simulink model "APPL_DriverFaultDetection"  (R2018b)
settings: configuration reference "CodeConfig_10_ms" (kept outside this file)
undefined symbols (not defined in the file): CAL_LockErrNoTime_30ms, CAL_ManualSwValid_90s, CAL_MotorHallInvalid_2s, CAL_MotorMaxRunTime_60s, CAL_MotorRelayErr_2s, CAL_MotorStall_750ms, D_DrSoftStopDef_B, D_DrSoftStopDef_F, D_DrSoftStopDef_H, D_DrSoftStopDef_L, D_Relay_DownBackFault, D_Relay_UpFrontFault, enSeatMoveCmd, FALSE, TRUE
libraries: DareLib x95, simulink x2
(part 1 of 3)
settings Model: Creator=Administrator  LastModifiedBy=Administrator
settings ConfigSetRef: SourceLocation=Base Workspace

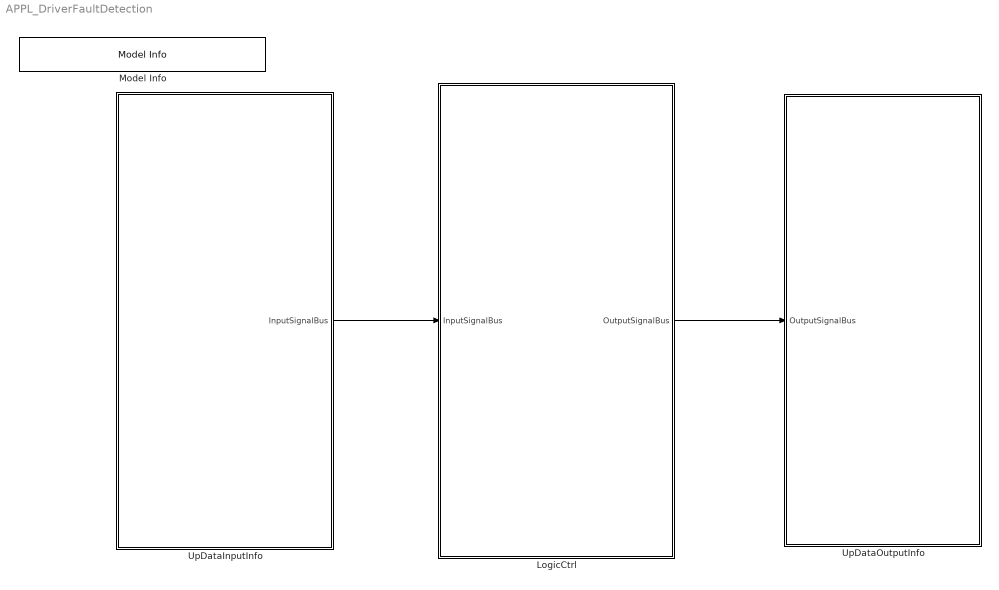
== system APPL_DriverFaultDetection ==
  LogicCtrl : Subsystem
  Model Info : simulink/Model-Wide Utilities/Model Info  Frame=on  DisplayStringWithTags=Version：%<ModelVersion>  HorizontalTextAlignment=Center  LeftAlignmentValue=0.5
  UpDataInputInfo : Subsystem  Priority=0  TreatAsAtomicUnit=on  RTWFileName=WiperCtrl
      settings: RTWSystemCode=Nonreusable function  RTWFcnNameOpts=Use subsystem name
  UpDataOutputInfo : Subsystem  Priority=2  TreatAsAtomicUnit=on  RTWFileName=WiperCtrl
      settings: RTWSystemCode=Nonreusable function  RTWFcnNameOpts=Use subsystem name
  wires:
  UpDataInputInfo/1(InputSignalBus) -> LogicCtrl/1(InputSignalBus)
  LogicCtrl/1(OutputSignalBus) -> UpDataOutputInfo/1(OutputSignalBus)

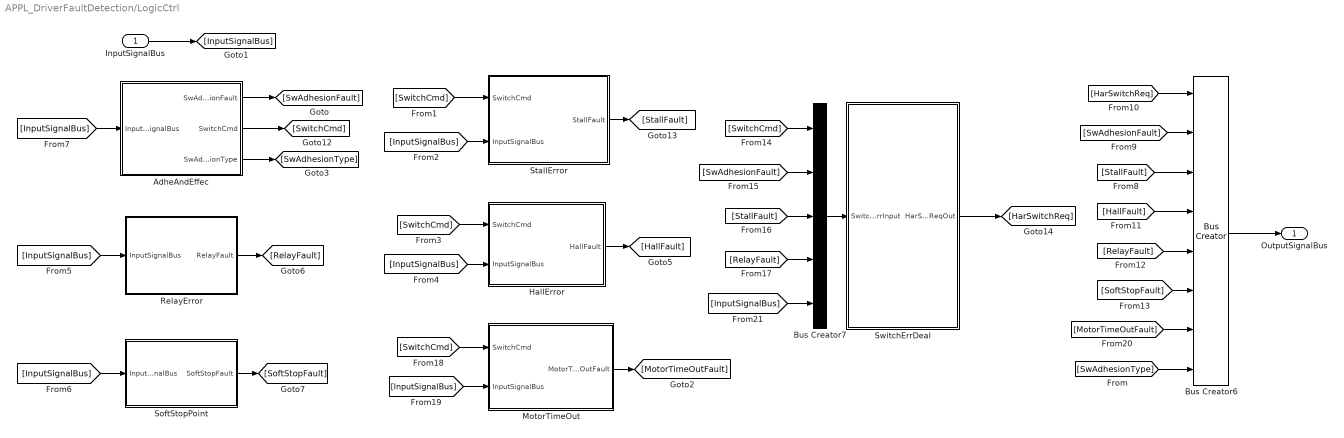
== system APPL_DriverFaultDetection/LogicCtrl ==
  InputSignalBus : Inport
  AdheAndEffec : Subsystem  Description=硬线开关粘连与有效检测
      settings: AttributesFormatString=%<Description>
  Bus Creator6 : BusCreator  Inputs=8
  Bus Creator7 : BusCreator  Inputs=5
  HallError : Subsystem  Description=电机霍尔故障检测
      settings: AttributesFormatString=%<Description>
  MotorTimeOut : Subsystem  Description=电机运行超时检测
      settings: AttributesFormatString=%<Description>
  RelayError : Subsystem  Description=继电器粘连故障检测
      settings: AttributesFormatString=%<Description>
  SoftStopPoint : Subsystem  Description=软止点检测
      settings: AttributesFormatString=%<Description>
  StallError : Subsystem  Description=电机堵转故障检测
      settings: AttributesFormatString=%<Description>
  SwitchErrDeal : Subsystem  Description=硬线开关故障处理
      settings: AttributesFormatString=%<Description>
  OutputSignalBus : Outport
  wires:
  InputSignalBus/1 -> [InputSignalBus]
  [StallFault] -> Bus Creator6/3
  [HallFault] -> Bus Creator6/4
  [SwAdhesionFault] -> Bus Creator6/2
  [RelayFault] -> Bus Creator6/5
  [HarSwitchReq] -> Bus Creator6/1
  [SoftStopFault] -> Bus Creator6/6
  Bus Creator6/1 -> OutputSignalBus/1
  [InputSignalBus] -> AdheAndEffec/1(InputSignalBus)
  AdheAndEffec/1(SwAdhesionFault) -> [SwAdhesionFault]
  AdheAndEffec/2(SwitchCmd) -> [SwitchCmd]
  [SwitchCmd] -> StallError/1(SwitchCmd)
  [InputSignalBus] -> StallError/2(InputSignalBus)
  StallError/1(StallFault) -> [StallFault]
  [SwitchCmd] -> HallError/1(SwitchCmd)
  [InputSignalBus] -> HallError/2(InputSignalBus)
  HallError/1(HallFault) -> [HallFault]
  [InputSignalBus] -> RelayError/1(InputSignalBus)
  RelayError/1(RelayFault) -> [RelayFault]
  SoftStopPoint/1(SoftStopFault) -> [SoftStopFault]
  [InputSignalBus] -> SoftStopPoint/1(InputSignalBus)
  SwitchErrDeal/1(HarSwitchReqOut) -> [HarSwitchReq]
  [SwitchCmd] -> Bus Creator7/1
  [StallFault] -> Bus Creator7/3
  [RelayFault] -> Bus Creator7/4
  [SwAdhesionFault] -> Bus Creator7/2
  Bus Creator7/1 -> SwitchErrDeal/1(SwitchErrInput)
  [SwitchCmd] -> MotorTimeOut/1(SwitchCmd)
  [InputSignalBus] -> MotorTimeOut/2(InputSignalBus)
  MotorTimeOut/1(MotorTimeOutFault) -> [MotorTimeOutFault]
  [MotorTimeOutFault] -> Bus Creator6/7
  [InputSignalBus] -> Bus Creator7/5
  AdheAndEffec/3(SwAdhesionType) -> [SwAdhesionType]
  [SwAdhesionType] -> Bus Creator6/8

== system APPL_DriverFaultDetection/UpDataInputInfo ==
  InputSignalProcess : Subsystem  Description=数据处理
      settings: AttributesFormatString=%<Description>  RTWSystemCode=Nonreusable function  RTWFcnNameOpts=Use subsystem name
  RTE_InputSignal : Subsystem  Description=接口自动生成  TreatAsAtomicUnit=on
      settings: AttributesFormatString=%<Description>  RTWSystemCode=Nonreusable function  RTWFcnNameOpts=Use subsystem name
  InputSignalBus : Outport
  wires:
  RTE_InputSignal/1(RTE_SignalBus) -> InputSignalProcess/1(RTE_SignalBus)
  InputSignalProcess/1(InputSignalBus) -> InputSignalBus/1  "InputSignalBus"

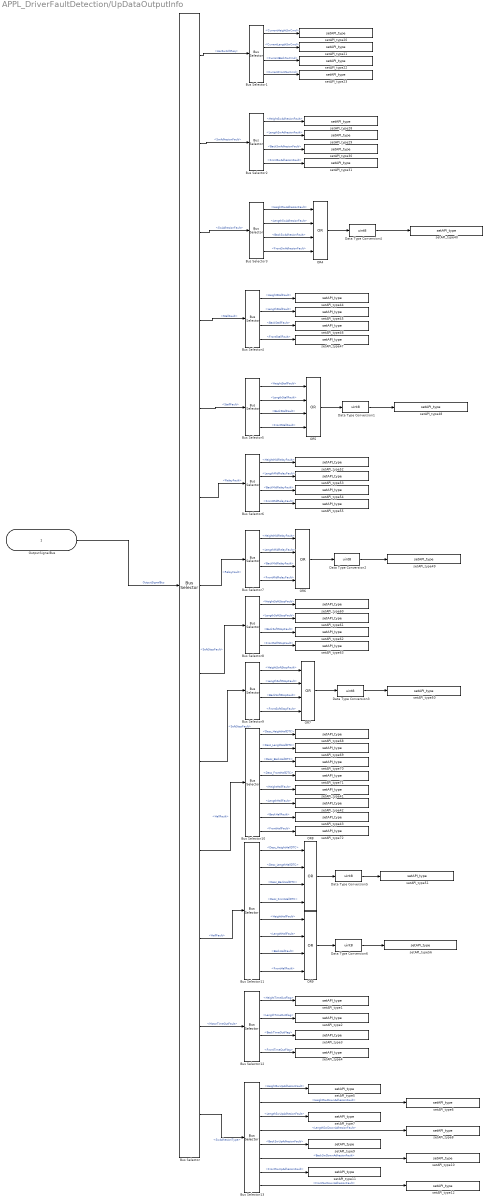
== system APPL_DriverFaultDetection/UpDataOutputInfo ==
  OutputSignalBus : Inport
  Bus Selector : BusSelector  OutputSignals=HarSwitchReq,SwAdhesionFault,SwAdhesionFault,StallFault,StallFault,RelayFault,RelayFault,SoftStopFault,SoftStopFault,HallFault,HallFault,MotorTimeOutFault,SwAdhesionType
  Bus Selector1 : BusSelector  OutputSignals=CurrentHeightSwCmd,CurrentLengthSwCmd,CurrentBackSwCmd,CurrentFrontSwCmd
  Bus Selector10 : BusSelector  OutputSignals=Desc_HeightHallDTC,Desc_LengthHallDTC,Desc_BackHallDTC,Desc_FrontHallDTC,HeightHallFault,LengthHallFault,BackHallFault,FrontHallFault
  Bus Selector11 : BusSelector  OutputSignals=Desc_HeightHallDTC,Desc_LengthHallDTC,Desc_BackHallDTC,Desc_FrontHallDTC,HeightHallFault,LengthHallFault,BackHallFault,FrontHallFault
  Bus Selector12 : BusSelector  OutputSignals=HeightTimeOutFlag,LengthTimeOutFlag,BackTimeOutFlag,FrontTimeOutFlag
  Bus Selector13 : BusSelector  OutputSignals=HeightSwUpAdhesionFault,HeightSwDownAdhesionFault,LengthSwUpAdhesionFault,LengthSwDownAdhesionFault,BackSwUpAdhesionFault,BackSwDownAdhesionFault,FrontSwUpAdhesionFault,FrontSwDownAdhesionFault
  Bus Selector2 : BusSelector  OutputSignals=HeightSwAdhesionFault,LengthSwAdhesionFault,BackSwAdhesionFault,FrontSwAdhesionFault
  Bus Selector3 : BusSelector  OutputSignals=HeightSwAdhesionFault,LengthSwAdhesionFault,BackSwAdhesionFault,FrontSwAdhesionFault
  Bus Selector4 : BusSelector  OutputSignals=HeightStallFault,LengthStallFault,BackStallFault,FrontStallFault
  Bus Selector5 : BusSelector  OutputSignals=HeightStallFault,LengthStallFault,BackStallFault,FrontStallFault
  Bus Selector6 : BusSelector  OutputSignals=HeightMidRelayFault,LengthMidRelayFault,BackMidRelayFault,FrontMidRelayFault
  Bus Selector7 : BusSelector  OutputSignals=HeightMidRelayFault,LengthMidRelayFault,BackMidRelayFault,FrontMidRelayFault
  Bus Selector8 : BusSelector  OutputSignals=HeightSoftStopFault,LengthSoftStopFault,BackSoftStopFault,FrontSoftStopFault
  Bus Selector9 : BusSelector  OutputSignals=HeightSoftStopFault,LengthSoftStopFault,BackSoftStopFault,FrontSoftStopFault
  Data Type Conversion{1..6} (6 alike) : DataTypeConversion  OutDataTypeStr=uint8
  OR{4..9} (6 alike) : Logic  Operator=OR  Inputs=4  AllPortsSameDT=off  OutDataTypeStr=boolean
  setAPI_type1 : DareLib/Dare/setAPI_type  g_funcname=Rte_SetVfb_DrHeightMotorTimeOutErr  g_param=""  g_type=uint8  g_size=-1
      settings: AttributesFormatString=%<g_funcname>  SourceProductName=Dare Library
  setAPI_type10 : DareLib/Dare/setAPI_type  g_funcname=Rte_SetVfb_DrBackSwitchAdheErr_Back  g_param=""  g_type=uint8  g_size=-1
      settings: AttributesFormatString=%<g_funcname>  SourceProductName=Dare Library
  setAPI_type11 : DareLib/Dare/setAPI_type  g_funcname=Rte_SetVfb_DrFrontSwitchAdheErr_ForWard  g_param=""  g_type=uint8  g_size=-1
      settings: AttributesFormatString=%<g_funcname>  SourceProductName=Dare Library
  setAPI_type12 : DareLib/Dare/setAPI_type  g_funcname=Rte_SetVfb_DrFrontSwitchAdheErr_Back  g_param=""  g_type=uint8  g_size=-1
      settings: AttributesFormatString=%<g_funcname>  SourceProductName=Dare Library
  setAPI_type2 : DareLib/Dare/setAPI_type  g_funcname=Rte_SetVfb_DrLengthMotorTimeOutErr  g_param=""  g_type=uint8  g_size=-1
      settings: AttributesFormatString=%<g_funcname>  SourceProductName=Dare Library
  setAPI_type20 : DareLib/Dare/setAPI_type  g_funcname=Rte_SetVfb_DrHeightSwitchCmd  g_param=""  g_type=uint8  g_enum=enSeatMoveCmd  g_size=-1
      settings: AttributesFormatString=%<g_funcname>  SourceProductName=Dare Library
  setAPI_type21 : DareLib/Dare/setAPI_type  g_funcname=Rte_SetVfb_DrLengthSwitchCmd  g_param=""  g_type=uint8  g_enum=enSeatMoveCmd  g_size=-1
      settings: AttributesFormatString=%<g_funcname>  SourceProductName=Dare Library
  setAPI_type22 : DareLib/Dare/setAPI_type  g_funcname=Rte_SetVfb_DrBackSwitchCmd  g_param=""  g_type=uint8  g_enum=enSeatMoveCmd  g_size=-1
      settings: AttributesFormatString=%<g_funcname>  SourceProductName=Dare Library
  setAPI_type23 : DareLib/Dare/setAPI_type  g_funcname=Rte_SetVfb_DrFrontSwitchCmd  g_param=""  g_type=uint8  g_enum=enSeatMoveCmd  g_size=-1
      settings: AttributesFormatString=%<g_funcname>  SourceProductName=Dare Library
  setAPI_type28 : DareLib/Dare/setAPI_type  g_funcname=Rte_SetVfb_DrHeightSwitchAdheErr  g_param=""  g_type=uint8  g_size=-1
      settings: AttributesFormatString=%<g_funcname>  SourceProductName=Dare Library
  setAPI_type29 : DareLib/Dare/setAPI_type  g_funcname=Rte_SetVfb_DrLengthSwitchAdheErr  g_param=""  g_type=uint8  g_size=-1
      settings: AttributesFormatString=%<g_funcname>  SourceProductName=Dare Library
  setAPI_type3 : DareLib/Dare/setAPI_type  g_funcname=Rte_SetVfb_DrBackMotorTimeOutErr  g_param=""  g_type=uint8  g_size=-1
      settings: AttributesFormatString=%<g_funcname>  SourceProductName=Dare Library
  setAPI_type30 : DareLib/Dare/setAPI_type  g_funcname=Rte_SetVfb_DrBackSwitchAdheErr  g_param=""  g_type=uint8  g_size=-1
      settings: AttributesFormatString=%<g_funcname>  SourceProductName=Dare Library
  setAPI_type31 : DareLib/Dare/setAPI_type  g_funcname=Rte_SetVfb_DrFrontSwitchAdheErr  g_param=""  g_type=uint8  g_size=-1
      settings: AttributesFormatString=%<g_funcname>  SourceProductName=Dare Library
  setAPI_type4 : DareLib/Dare/setAPI_type  g_funcname=Rte_SetVfb_DrFrontMotorTimeOutErr  g_param=""  g_type=uint8  g_size=-1
      settings: AttributesFormatString=%<g_funcname>  SourceProductName=Dare Library
  setAPI_type40 : DareLib/Dare/setAPI_type  g_funcname=Rte_SetVfb_DrAnyoneSwitchAdheErr  g_param=""  g_type=uint8  g_size=-1
      settings: AttributesFormatString=%<g_funcname>  SourceProductName=Dare Library
  setAPI_type41 : DareLib/Dare/setAPI_type  g_funcname=Rte_SetVfb_DrHeightHallErr  g_param=""  g_type=uint8  g_size=-1
      settings: AttributesFormatString=%<g_funcname>  SourceProductName=Dare Library
  setAPI_type42 : DareLib/Dare/setAPI_type  g_funcname=Rte_SetVfb_DrLengthHallErr  g_param=""  g_type=uint8  g_size=-1
      settings: AttributesFormatString=%<g_funcname>  SourceProductName=Dare Library
  setAPI_type43 : DareLib/Dare/setAPI_type  g_funcname=Rte_SetVfb_DrBackHallErr  g_param=""  g_type=uint8  g_size=-1
      settings: AttributesFormatString=%<g_funcname>  SourceProductName=Dare Library
  setAPI_type44 : DareLib/Dare/setAPI_type  g_funcname=Rte_SetVfb_DrHeightStallErr  g_param=""  g_type=uint8  g_size=-1
      settings: AttributesFormatString=%<g_funcname>  SourceProductName=Dare Library
  setAPI_type45 : DareLib/Dare/setAPI_type  g_funcname=Rte_SetVfb_DrLengthStallErr  g_param=""  g_type=uint8  g_size=-1
      settings: AttributesFormatString=%<g_funcname>  SourceProductName=Dare Library
  setAPI_type46 : DareLib/Dare/setAPI_type  g_funcname=Rte_SetVfb_DrBackStallErr  g_param=""  g_type=uint8  g_size=-1
      settings: AttributesFormatString=%<g_funcname>  SourceProductName=Dare Library
  setAPI_type47 : DareLib/Dare/setAPI_type  g_funcname=Rte_SetVfb_DrFrontStallErr  g_param=""  g_type=uint8  g_size=-1
      settings: AttributesFormatString=%<g_funcname>  SourceProductName=Dare Library
  setAPI_type48 : DareLib/Dare/setAPI_type  g_funcname=Rte_SetVfb_DrAnyoneStallErr  g_param=""  g_type=uint8  g_size=-1
      settings: AttributesFormatString=%<g_funcname>  SourceProductName=Dare Library
  setAPI_type49 : DareLib/Dare/setAPI_type  g_funcname=Rte_SetVfb_DrAnyoneRelayAdheErr  g_param=""  g_type=uint8  g_size=-1
      settings: AttributesFormatString=%<g_funcname>  SourceProductName=Dare Library
  setAPI_type5 : DareLib/Dare/setAPI_type  g_funcname=Rte_SetVfb_DrHeightSwitchAdheErr_ForWard  g_param=""  g_type=uint8  g_size=-1
      settings: AttributesFormatString=%<g_funcname>  SourceProductName=Dare Library
  setAPI_type50 : DareLib/Dare/setAPI_type  g_funcname=Rte_SetVfb_DrAnyoneSoftStopErr  g_param=""  g_type=uint8  g_size=-1
      settings: AttributesFormatString=%<g_funcname>  SourceProductName=Dare Library
  setAPI_type51 : DareLib/Dare/setAPI_type  g_funcname=Rte_SetVfb_DrAnyoneDTCHallErr  g_param=""  g_type=uint8  g_size=-1
      settings: AttributesFormatString=%<g_funcname>  SourceProductName=Dare Library
  setAPI_type52 : DareLib/Dare/setAPI_type  g_funcname=Rte_SetVfb_DrHeightRelayAdheErr  g_param=""  g_type=uint8  g_size=-1
      settings: AttributesFormatString=%<g_funcname>  SourceProductName=Dare Library
  setAPI_type53 : DareLib/Dare/setAPI_type  g_funcname=Rte_SetVfb_DrLengthRelayAdheErr  g_param=""  g_type=uint8  g_size=-1
      settings: AttributesFormatString=%<g_funcname>  SourceProductName=Dare Library
  setAPI_type54 : DareLib/Dare/setAPI_type  g_funcname=Rte_SetVfb_DrBackRelayAdheErr  g_param=""  g_type=uint8  g_size=-1
      settings: AttributesFormatString=%<g_funcname>  SourceProductName=Dare Library
  setAPI_type55 : DareLib/Dare/setAPI_type  g_funcname=Rte_SetVfb_DrFrontRelayAdheErr  g_param=""  g_type=uint8  g_size=-1
      settings: AttributesFormatString=%<g_funcname>  SourceProductName=Dare Library
  setAPI_type56 : DareLib/Dare/setAPI_type  g_funcname=Rte_SetVfb_DrAnyoneHallErr  g_param=""  g_type=uint8  g_size=-1
      settings: AttributesFormatString=%<g_funcname>  SourceProductName=Dare Library
  setAPI_type6 : DareLib/Dare/setAPI_type  g_funcname=Rte_SetVfb_DrHeightSwitchAdheErr_Back  g_param=""  g_type=uint8  g_size=-1
      settings: AttributesFormatString=%<g_funcname>  SourceProductName=Dare Library
  setAPI_type60 : DareLib/Dare/setAPI_type  g_funcname=Rte_SetVfb_DrHeightSoftStopErr  g_param=""  g_type=uint8  g_size=-1
      settings: AttributesFormatString=%<g_funcname>  SourceProductName=Dare Library
  setAPI_type61 : DareLib/Dare/setAPI_type  g_funcname=Rte_SetVfb_DrLengthSoftStopErr  g_param=""  g_type=uint8  g_size=-1
      settings: AttributesFormatString=%<g_funcname>  SourceProductName=Dare Library
  setAPI_type62 : DareLib/Dare/setAPI_type  g_funcname=Rte_SetVfb_DrBackSoftStopErr  g_param=""  g_type=uint8  g_size=-1
      settings: AttributesFormatString=%<g_funcname>  SourceProductName=Dare Library
  setAPI_type63 : DareLib/Dare/setAPI_type  g_funcname=Rte_SetVfb_DrFrontSoftStopErr  g_param=""  g_type=uint8  g_size=-1
      settings: AttributesFormatString=%<g_funcname>  SourceProductName=Dare Library
  setAPI_type68 : DareLib/Dare/setAPI_type  g_funcname=Rte_SetVfb_DrHeightDTCHallErr  g_param=""  g_type=uint8  g_size=-1
      settings: AttributesFormatString=%<g_funcname>  SourceProductName=Dare Library
  setAPI_type69 : DareLib/Dare/setAPI_type  g_funcname=Rte_SetVfb_DrLengthDTCHallErr  g_param=""  g_type=uint8  g_size=-1
      settings: AttributesFormatString=%<g_funcname>  SourceProductName=Dare Library
  setAPI_type7 : DareLib/Dare/setAPI_type  g_funcname=Rte_SetVfb_DrLengthSwitchAdheErr_ForWard  g_param=""  g_type=uint8  g_size=-1
      settings: AttributesFormatString=%<g_funcname>  SourceProductName=Dare Library
  setAPI_type70 : DareLib/Dare/setAPI_type  g_funcname=Rte_SetVfb_DrBackDTCHallErr  g_param=""  g_type=uint8  g_size=-1
      settings: AttributesFormatString=%<g_funcname>  SourceProductName=Dare Library
  setAPI_type71 : DareLib/Dare/setAPI_type  g_funcname=Rte_SetVfb_DrFrontDTCHallErr  g_param=""  g_type=uint8  g_size=-1
      settings: AttributesFormatString=%<g_funcname>  SourceProductName=Dare Library
  setAPI_type72 : DareLib/Dare/setAPI_type  g_funcname=Rte_SetVfb_DrFrontHallErr  g_param=""  g_type=uint8  g_size=-1
      settings: AttributesFormatString=%<g_funcname>  SourceProductName=Dare Library
  setAPI_type8 : DareLib/Dare/setAPI_type  g_funcname=Rte_SetVfb_DrLengthSwitchAdheErr_Back  g_param=""  g_type=uint8  g_size=-1
      settings: AttributesFormatString=%<g_funcname>  SourceProductName=Dare Library
  setAPI_type9 : DareLib/Dare/setAPI_type  g_funcname=Rte_SetVfb_DrBackSwitchAdheErr_ForWard  g_param=""  g_type=uint8  g_size=-1
      settings: AttributesFormatString=%<g_funcname>  SourceProductName=Dare Library
  wires:
  OutputSignalBus/1 -> Bus Selector/1  "OutputSignalBus"
  Bus Selector/1 -> Bus Selector1/1  "<HarSwitchReq>"
  Bus Selector1/1 -> setAPI_type20/1  "<CurrentHeightSwCmd>"
  Bus Selector1/2 -> setAPI_type21/1  "<CurrentLengthSwCmd>"
  Bus Selector1/3 -> setAPI_type22/1  "<CurrentBackSwCmd>"
  Bus Selector1/4 -> setAPI_type23/1  "<CurrentFrontSwCmd>"
  Bus Selector/2 -> Bus Selector2/1  "<SwAdhesionFault>"
  Bus Selector2/1 -> setAPI_type28/1  "<HeightSwAdhesionFault>"
  Bus Selector2/2 -> setAPI_type29/1  "<LengthSwAdhesionFault>"
  Bus Selector2/3 -> setAPI_type30/1  "<BackSwAdhesionFault>"
  Bus Selector2/4 -> setAPI_type31/1  "<FrontSwAdhesionFault>"
  Bus Selector4/1 -> setAPI_type44/1  "<HeightStallFault>"
  Bus Selector4/2 -> setAPI_type45/1  "<LengthStallFault>"
  Bus Selector4/3 -> setAPI_type46/1  "<BackStallFault>"
  Bus Selector4/4 -> setAPI_type47/1  "<FrontStallFault>"
  Bus Selector6/1 -> setAPI_type52/1  "<HeightMidRelayFault>"
  Bus Selector6/2 -> setAPI_type53/1  "<LengthMidRelayFault>"
  Bus Selector6/3 -> setAPI_type54/1  "<BackMidRelayFault>"
  Bus Selector6/4 -> setAPI_type55/1  "<FrontMidRelayFault>"
  Bus Selector7/4 -> OR6/4  "<FrontMidRelayFault>"
  Bus Selector7/3 -> OR6/3  "<BackMidRelayFault>"
  Bus Selector7/2 -> OR6/2  "<LengthMidRelayFault>"
  Bus Selector7/1 -> OR6/1  "<HeightMidRelayFault>"
  Bus Selector8/1 -> setAPI_type60/1  "<HeightSoftStopFault>"
  Bus Selector8/2 -> setAPI_type61/1  "<LengthSoftStopFault>"
  Bus Selector8/3 -> setAPI_type62/1  "<BackSoftStopFault>"
  Bus Selector8/4 -> setAPI_type63/1  "<FrontSoftStopFault>"
  Bus Selector9/4 -> OR7/4  "<FrontSoftStopFault>"
  Bus Selector9/3 -> OR7/3  "<BackSoftStopFault>"
  Bus Selector9/2 -> OR7/2  "<LengthSoftStopFault>"
  Bus Selector9/1 -> OR7/1  "<HeightSoftStopFault>"
  Bus Selector3/1 -> OR4/1  "<HeightSwAdhesionFault>"
  Bus Selector3/2 -> OR4/2  "<LengthSwAdhesionFault>"
  Bus Selector3/3 -> OR4/3  "<BackSwAdhesionFault>"
  Bus Selector3/4 -> OR4/4  "<FrontSwAdhesionFault>"
  Bus Selector/3 -> Bus Selector3/1  "<SwAdhesionFault>"
  Bus Selector/4 -> Bus Selector4/1  "<StallFault>"
  Bus Selector/5 -> Bus Selector5/1  "<StallFault>"
  Bus Selector/6 -> Bus Selector6/1  "<RelayFault>"
  Bus Selector/7 -> Bus Selector7/1  "<RelayFault>"
  Bus Selector/8 -> Bus Selector8/1  "<SoftStopFault>"
  Bus Selector/9 -> Bus Selector9/1  "<SoftStopFault>"
  Bus Selector/10 -> Bus Selector10/1  "<HallFault>"
  Bus Selector10/1 -> setAPI_type68/1  "<Desc_HeightHallDTC>"
  Bus Selector10/2 -> setAPI_type69/1  "<Desc_LengthHallDTC>"
  Bus Selector10/3 -> setAPI_type70/1  "<Desc_BackHallDTC>"
  Bus Selector10/4 -> setAPI_type71/1  "<Desc_FrontHallDTC>"
  Bus Selector10/5 -> setAPI_type41/1  "<HeightHallFault>"
  Bus Selector10/6 -> setAPI_type42/1  "<LengthHallFault>"
  Bus Selector10/7 -> setAPI_type43/1  "<BackHallFault>"
  Bus Selector10/8 -> setAPI_type72/1  "<FrontHallFault>"
  Bus Selector/11 -> Bus Selector11/1  "<HallFault>"
  Bus Selector5/1 -> OR5/1  "<HeightStallFault>"
  Bus Selector5/2 -> OR5/2  "<LengthStallFault>"
  Bus Selector5/3 -> OR5/3  "<BackStallFault>"
  Bus Selector5/4 -> OR5/4  "<FrontStallFault>"
  Bus Selector11/1 -> OR8/1  "<Desc_HeightHallDTC>"
  Bus Selector11/2 -> OR8/2  "<Desc_LengthHallDTC>"
  Bus Selector11/3 -> OR8/3  "<Desc_BackHallDTC>"
  Bus Selector11/4 -> OR8/4  "<Desc_FrontHallDTC>"
  Bus Selector11/8 -> OR9/4  "<FrontHallFault>"
  Bus Selector11/7 -> OR9/3  "<BackHallFault>"
  Bus Selector11/6 -> OR9/2  "<LengthHallFault>"
  Bus Selector11/5 -> OR9/1  "<HeightHallFault>"
  Data Type Conversion4/1 -> setAPI_type40/1
  OR4/1 -> Data Type Conversion4/1
  OR5/1 -> Data Type Conversion1/1
  Data Type Conversion1/1 -> setAPI_type48/1
  OR6/1 -> Data Type Conversion2/1
  Data Type Conversion2/1 -> setAPI_type49/1
  OR7/1 -> Data Type Conversion3/1
  Data Type Conversion3/1 -> setAPI_type50/1
  OR8/1 -> Data Type Conversion5/1
  OR9/1 -> Data Type Conversion6/1
  Data Type Conversion6/1 -> setAPI_type56/1
  Data Type Conversion5/1 -> setAPI_type51/1
  Bus Selector/12 -> Bus Selector12/1  "<MotorTimeOutFault>"
  Bus Selector12/2 -> setAPI_type2/1  "<LengthTimeOutFlag>"
  Bus Selector12/3 -> setAPI_type3/1  "<BackTimeOutFlag>"
  Bus Selector12/1 -> setAPI_type1/1  "<HeightTimeOutFlag>"
  Bus Selector12/4 -> setAPI_type4/1  "<FrontTimeOutFlag>"
  Bus Selector13/1 -> setAPI_type5/1  "<HeightSwUpAdhesionFault>"
  Bus Selector13/2 -> setAPI_type6/1  "<HeightSwDownAdhesionFault>"
  Bus Selector13/3 -> setAPI_type7/1  "<LengthSwUpAdhesionFault>"
  Bus Selector13/4 -> setAPI_type8/1  "<LengthSwDownAdhesionFault>"
  Bus Selector13/5 -> setAPI_type9/1  "<BackSwUpAdhesionFault>"
  Bus Selector13/6 -> setAPI_type10/1  "<BackSwDownAdhesionFault>"
  Bus Selector13/7 -> setAPI_type11/1  "<FrontSwUpAdhesionFault>"
  Bus Selector13/8 -> setAPI_type12/1  "<FrontSwDownAdhesionFault>"
  Bus Selector/13 -> Bus Selector13/1  "<SwAdhesionType>"

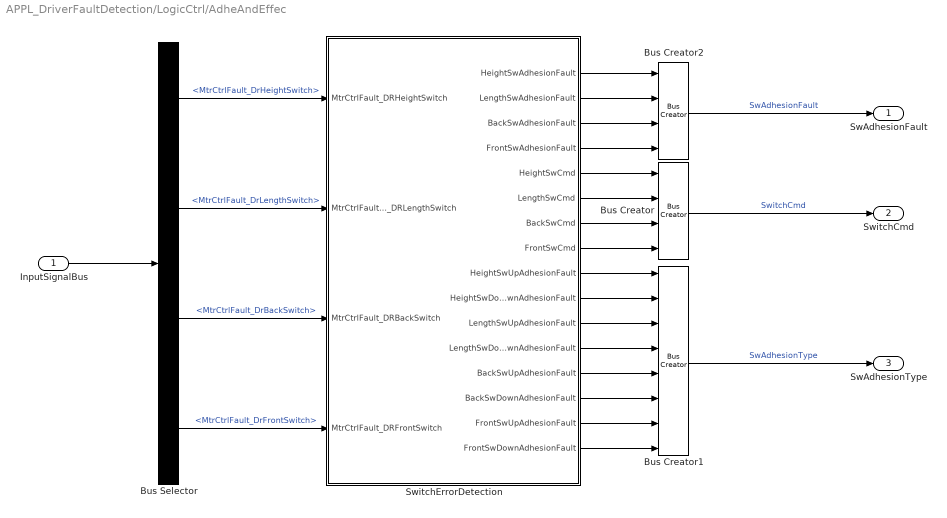
== system APPL_DriverFaultDetection/LogicCtrl/AdheAndEffec ==
  InputSignalBus : Inport
  Bus Creator : BusCreator  Inputs=4
  Bus Creator1 : BusCreator  Inputs=8
  Bus Creator2 : BusCreator  Inputs=4
  Bus Selector : BusSelector  OutputSignals=SwitchInCmd.MtrCtrlFault_DrHeightSwitch,SwitchInCmd.MtrCtrlFault_DrLengthSwitch,SwitchInCmd.MtrCtrlFault_DrBackSwitch,SwitchInCmd.MtrCtrlFault_DrFrontSwitch
  SwitchErrorDetection : Stateflow chart  TreatAsAtomicUnit=on
  SwAdhesionFault : Outport
  SwitchCmd : Outport  Port=2
  SwAdhesionType : Outport  Port=3
  wires:
  Bus Selector/2 -> SwitchErrorDetection/2(MtrCtrlFault_DRLengthSwitch)  "<MtrCtrlFault_DrLengthSwitch>"
  Bus Selector/1 -> SwitchErrorDetection/1(MtrCtrlFault_DRHeightSwitch)  "<MtrCtrlFault_DrHeightSwitch>"
  SwitchErrorDetection/3(BackSwAdhesionFault) -> Bus Creator2/3
  Bus Selector/4 -> SwitchErrorDetection/4(MtrCtrlFault_DRFrontSwitch)  "<MtrCtrlFault_DrFrontSwitch>"
  SwitchErrorDetection/2(LengthSwAdhesionFault) -> Bus Creator2/2
  Bus Selector/3 -> SwitchErrorDetection/3(MtrCtrlFault_DRBackSwitch)  "<MtrCtrlFault_DrBackSwitch>"
  SwitchErrorDetection/7(BackSwCmd) -> Bus Creator/3
  SwitchErrorDetection/6(LengthSwCmd) -> Bus Creator/2
  SwitchErrorDetection/8(FrontSwCmd) -> Bus Creator/4
  SwitchErrorDetection/5(HeightSwCmd) -> Bus Creator/1
  SwitchErrorDetection/1(HeightSwAdhesionFault) -> Bus Creator2/1
  SwitchErrorDetection/4(FrontSwAdhesionFault) -> Bus Creator2/4
  InputSignalBus/1 -> Bus Selector/1
  Bus Creator2/1 -> SwAdhesionFault/1  "SwAdhesionFault"
  Bus Creator/1 -> SwitchCmd/1  "SwitchCmd"
  SwitchErrorDetection/9(HeightSwUpAdhesionFault) -> Bus Creator1/1
  SwitchErrorDetection/10(HeightSwDownAdhesionFault) -> Bus Creator1/2
  SwitchErrorDetection/11(LengthSwUpAdhesionFault) -> Bus Creator1/3
  SwitchErrorDetection/12(LengthSwDownAdhesionFault) -> Bus Creator1/4
  SwitchErrorDetection/13(BackSwUpAdhesionFault) -> Bus Creator1/5
  SwitchErrorDetection/14(BackSwDownAdhesionFault) -> Bus Creator1/6
  SwitchErrorDetection/15(FrontSwUpAdhesionFault) -> Bus Creator1/7
  SwitchErrorDetection/16(FrontSwDownAdhesionFault) -> Bus Creator1/8
  Bus Creator1/1 -> SwAdhesionType/1  "SwAdhesionType"

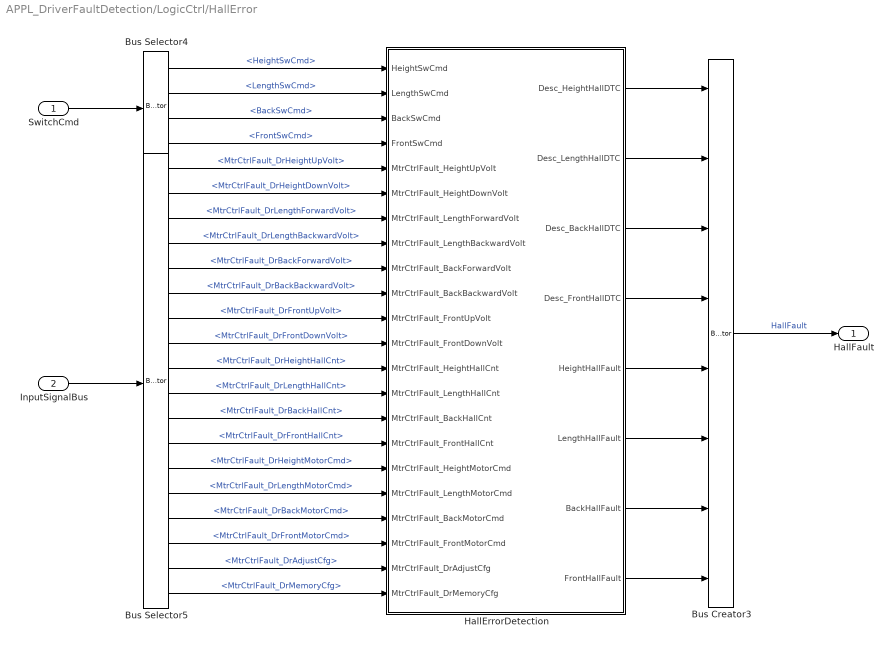
== system APPL_DriverFaultDetection/LogicCtrl/HallError ==
  SwitchCmd : Inport
  InputSignalBus : Inport  Port=2
  Bus Creator3 : BusCreator  Inputs=8
  Bus Selector4 : BusSelector  OutputSignals=HeightSwCmd,LengthSwCmd,BackSwCmd,FrontSwCmd
  Bus Selector5 : BusSelector  OutputSignals=RelayVolt.MtrCtrlFault_DrHeightUpVolt,RelayVolt.MtrCtrlFault_DrHeightDownVolt,RelayVolt.MtrCtrlFault_DrLengthForwardVolt,RelayVolt.MtrCtrlFault_DrLengthBackwardVolt,RelayVolt.MtrCtrlFault_DrBackForwardVolt,RelayVolt.MtrCtrlFault_DrBackBackwardVolt,RelayVolt.MtrCtrlFault_DrFrontUpVolt,RelayVolt.MtrCtrlFault_DrFrontDownVolt,HallCnt.MtrCtrlFault_DrHeightHallCnt,HallCnt.MtrCtrlFault_DrLengthHallCnt,HallCnt.MtrCtrlFault_DrBackHallCnt,HallCnt.MtrCtrlFault_DrFrontHallCnt,MotorCmd.MtrCtrlFault_DrHeightMotorCmd,MotorCmd.MtrCtrlFault_DrLengthMotorCmd,MotorCmd.MtrCtrlFault_DrBackMotorCmd,MotorCmd.MtrCtrlFault_DrFrontMotorCmd,Config.MtrCtrlFault_DrAdjustCfg,Config.MtrCtrlFault_DrMemoryCfg
  HallErrorDetection : Stateflow chart  TreatAsAtomicUnit=on
  HallFault : Outport
  wires:
  Bus Selector5/12 -> HallErrorDetection/16(MtrCtrlFault_FrontHallCnt)  "<MtrCtrlFault_DrFrontHallCnt>"
  Bus Selector5/14 -> HallErrorDetection/18(MtrCtrlFault_LengthMotorCmd)  "<MtrCtrlFault_DrLengthMotorCmd>"
  SwitchCmd/1 -> Bus Selector4/1
  Bus Selector5/13 -> HallErrorDetection/17(MtrCtrlFault_HeightMotorCmd)  "<MtrCtrlFault_DrHeightMotorCmd>"
  Bus Selector5/9 -> HallErrorDetection/13(MtrCtrlFault_HeightHallCnt)  "<MtrCtrlFault_DrHeightHallCnt>"
  Bus Selector5/8 -> HallErrorDetection/12(MtrCtrlFault_FrontDownVolt)  "<MtrCtrlFault_DrFrontDownVolt>"
  Bus Selector5/11 -> HallErrorDetection/15(MtrCtrlFault_BackHallCnt)  "<MtrCtrlFault_DrBackHallCnt>"
  Bus Selector5/6 -> HallErrorDetection/10(MtrCtrlFault_BackBackwardVolt)  "<MtrCtrlFault_DrBackBackwardVolt>"
  Bus Selector5/1 -> HallErrorDetection/5(MtrCtrlFault_HeightUpVolt)  "<MtrCtrlFault_DrHeightUpVolt>"
  Bus Selector4/3 -> HallErrorDetection/3(BackSwCmd)  "<BackSwCmd>"
  Bus Selector5/7 -> HallErrorDetection/11(MtrCtrlFault_FrontUpVolt)  "<MtrCtrlFault_DrFrontUpVolt>"
  InputSignalBus/1 -> Bus Selector5/1
  Bus Selector5/16 -> HallErrorDetection/20(MtrCtrlFault_FrontMotorCmd)  "<MtrCtrlFault_DrFrontMotorCmd>"
  Bus Selector4/1 -> HallErrorDetection/1(HeightSwCmd)  "<HeightSwCmd>"
  Bus Selector5/10 -> HallErrorDetection/14(MtrCtrlFault_LengthHallCnt)  "<MtrCtrlFault_DrLengthHallCnt>"
  Bus Selector4/2 -> HallErrorDetection/2(LengthSwCmd)  "<LengthSwCmd>"
  Bus Selector5/4 -> HallErrorDetection/8(MtrCtrlFault_LengthBackwardVolt)  "<MtrCtrlFault_DrLengthBackwardVolt>"
  HallErrorDetection/4(Desc_FrontHallDTC) -> Bus Creator3/4
  HallErrorDetection/3(Desc_BackHallDTC) -> Bus Creator3/3
  Bus Creator3/1 -> HallFault/1  "HallFault"
  HallErrorDetection/7(BackHallFault) -> Bus Creator3/7
  HallErrorDetection/5(HeightHallFault) -> Bus Creator3/5
  Bus Selector5/2 -> HallErrorDetection/6(MtrCtrlFault_HeightDownVolt)  "<MtrCtrlFault_DrHeightDownVolt>"
  HallErrorDetection/6(LengthHallFault) -> Bus Creator3/6
  Bus Selector5/3 -> HallErrorDetection/7(MtrCtrlFault_LengthForwardVolt)  "<MtrCtrlFault_DrLengthForwardVolt>"
  HallErrorDetection/1(Desc_HeightHallDTC) -> Bus Creator3/1
  Bus Selector5/15 -> HallErrorDetection/19(MtrCtrlFault_BackMotorCmd)  "<MtrCtrlFault_DrBackMotorCmd>"
  HallErrorDetection/2(Desc_LengthHallDTC) -> Bus Creator3/2
  Bus Selector4/4 -> HallErrorDetection/4(FrontSwCmd)  "<FrontSwCmd>"
  Bus Selector5/5 -> HallErrorDetection/9(MtrCtrlFault_BackForwardVolt)  "<MtrCtrlFault_DrBackForwardVolt>"
  HallErrorDetection/8(FrontHallFault) -> Bus Creator3/8
  Bus Selector5/17 -> HallErrorDetection/21(MtrCtrlFault_DrAdjustCfg)  "<MtrCtrlFault_DrAdjustCfg>"
  Bus Selector5/18 -> HallErrorDetection/22(MtrCtrlFault_DrMemoryCfg)  "<MtrCtrlFault_DrMemoryCfg>"

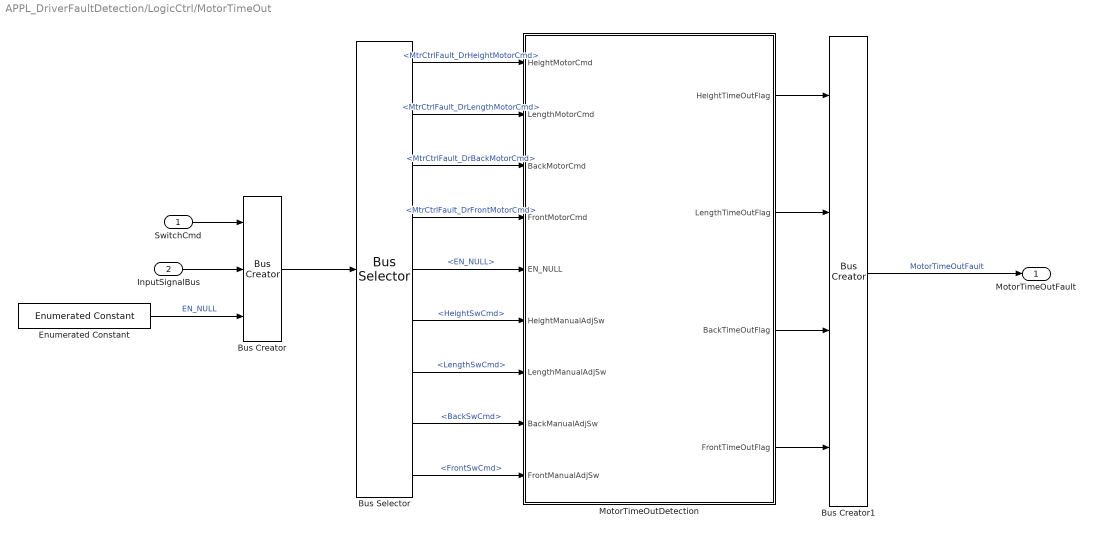
== system APPL_DriverFaultDetection/LogicCtrl/MotorTimeOut ==
  SwitchCmd : Inport
  InputSignalBus : Inport  Port=2
  Bus Creator : BusCreator  Inputs=3
  Bus Creator1 : BusCreator  Inputs=4
  Bus Selector : BusSelector  OutputSignals=InputSignalBus.MotorCmd.MtrCtrlFault_DrHeightMotorCmd,InputSignalBus.MotorCmd.MtrCtrlFault_DrLengthMotorCmd,InputSignalBus.MotorCmd.MtrCtrlFault_DrBackMotorCmd,InputSignalBus.MotorCmd.MtrCtrlFault_DrFrontMotorCmd,EN_NULL,SwitchCmd.HeightSwCmd,SwitchCmd.LengthSwCmd,SwitchCmd.BackSwCmd,SwitchCmd.FrontSwCmd
  Enumerated Constant : simulink/Sources/Enumerated Constant  OutDataTypeStr=Enum: enSeatMoveCmd  Value=enSeatMoveCmd.EN_NULL  SampleTime=inf
      settings: SourceProductName=Simulink
  MotorTimeOutDetection : Stateflow chart  TreatAsAtomicUnit=on
  MotorTimeOutFault : Outport
  wires:
  SwitchCmd/1 -> Bus Creator/1
  Bus Creator/1 -> Bus Selector/1
  InputSignalBus/1 -> Bus Creator/2
  Enumerated Constant/1 -> Bus Creator/3  "EN_NULL"
  Bus Selector/1 -> MotorTimeOutDetection/1(HeightMotorCmd)  "<MtrCtrlFault_DrHeightMotorCmd>"
  Bus Selector/2 -> MotorTimeOutDetection/2(LengthMotorCmd)  "<MtrCtrlFault_DrLengthMotorCmd>"
  Bus Selector/3 -> MotorTimeOutDetection/3(BackMotorCmd)  "<MtrCtrlFault_DrBackMotorCmd>"
  Bus Selector/4 -> MotorTimeOutDetection/4(FrontMotorCmd)  "<MtrCtrlFault_DrFrontMotorCmd>"
  Bus Selector/5 -> MotorTimeOutDetection/5(EN_NULL)  "<EN_NULL>"
  Bus Selector/6 -> MotorTimeOutDetection/6(HeightManualAdjSw)  "<HeightSwCmd>"
  Bus Selector/7 -> MotorTimeOutDetection/7(LengthManualAdjSw)  "<LengthSwCmd>"
  Bus Selector/8 -> MotorTimeOutDetection/8(BackManualAdjSw)  "<BackSwCmd>"
  Bus Selector/9 -> MotorTimeOutDetection/9(FrontManualAdjSw)  "<FrontSwCmd>"
  Bus Creator1/1 -> MotorTimeOutFault/1  "MotorTimeOutFault"
  MotorTimeOutDetection/4(FrontTimeOutFlag) -> Bus Creator1/4
  MotorTimeOutDetection/3(BackTimeOutFlag) -> Bus Creator1/3
  MotorTimeOutDetection/2(LengthTimeOutFlag) -> Bus Creator1/2
  MotorTimeOutDetection/1(HeightTimeOutFlag) -> Bus Creator1/1

== system APPL_DriverFaultDetection/LogicCtrl/RelayError ==
  InputSignalBus : Inport
  Bus Creator4 : BusCreator  Inputs=4
  Bus Selector6 : BusSelector  OutputSignals=RelayVolt.MtrCtrlFault_DrHeightUpVolt,RelayVolt.MtrCtrlFault_DrHeightDownVolt,RelayVolt.MtrCtrlFault_DrLengthForwardVolt,RelayVolt.MtrCtrlFault_DrLengthBackwardVolt,RelayVolt.MtrCtrlFault_DrBackForwardVolt,RelayVolt.MtrCtrlFault_DrBackBackwardVolt,RelayVolt.MtrCtrlFault_DrFrontUpVolt,RelayVolt.MtrCtrlFault_DrFrontDownVolt,MotorCmd.MtrCtrlFault_DrHeightMotorCmd,MotorCmd.MtrCtrlFault_DrLengthMotorCmd,MotorCmd.MtrCtrlFault_DrBackMotorCmd,MotorCmd.MtrCtrlFault_DrFrontMotorCmd
  MidRelayErrorDetection : Stateflow chart  TreatAsAtomicUnit=on
  RelayFault : Outport
  wires:
  Bus Selector6/9 -> MidRelayErrorDetection/9(MtrCtrlFault_HeightMotorCmd)  "<MtrCtrlFault_DrHeightMotorCmd>"
  Bus Selector6/2 -> MidRelayErrorDetection/2(MtrCtrlFault_HeightDownVolt)  "<MtrCtrlFault_DrHeightDownVolt>"
  Bus Selector6/7 -> MidRelayErrorDetection/7(MtrCtrlFault_FrontUpVolt)  "<MtrCtrlFault_DrFrontUpVolt>"
  Bus Selector6/10 -> MidRelayErrorDetection/10(MtrCtrlFault_LengthMotorCmd)  "<MtrCtrlFault_DrLengthMotorCmd>"
  Bus Selector6/11 -> MidRelayErrorDetection/11(MtrCtrlFault_BackMotorCmd)  "<MtrCtrlFault_DrBackMotorCmd>"
  MidRelayErrorDetection/4(FrontMidRelayFault) -> Bus Creator4/4
  Bus Selector6/1 -> MidRelayErrorDetection/1(MtrCtrlFault_HeightUpVolt)  "<MtrCtrlFault_DrHeightUpVolt>"
  Bus Selector6/8 -> MidRelayErrorDetection/8(MtrCtrlFault_FrontDownVolt)  "<MtrCtrlFault_DrFrontDownVolt>"
  Bus Selector6/3 -> MidRelayErrorDetection/3(MtrCtrlFault_LengthForwardVolt)  "<MtrCtrlFault_DrLengthForwardVolt>"
  MidRelayErrorDetection/2(LengthMidRelayFault) -> Bus Creator4/2
  InputSignalBus/1 -> Bus Selector6/1
  Bus Selector6/5 -> MidRelayErrorDetection/5(MtrCtrlFault_BackForwardVolt)  "<MtrCtrlFault_DrBackForwardVolt>"
  MidRelayErrorDetection/3(BackMidRelayFault) -> Bus Creator4/3
  Bus Selector6/12 -> MidRelayErrorDetection/12(MtrCtrlFault_FrontMotorCmd)  "<MtrCtrlFault_DrFrontMotorCmd>"
  Bus Selector6/6 -> MidRelayErrorDetection/6(MtrCtrlFault_BackBackwardVolt)  "<MtrCtrlFault_DrBackBackwardVolt>"
  Bus Selector6/4 -> MidRelayErrorDetection/4(MtrCtrlFault_LengthBackwardVolt)  "<MtrCtrlFault_DrLengthBackwardVolt>"
  MidRelayErrorDetection/1(HeightMidRelayFault) -> Bus Creator4/1
  Bus Creator4/1 -> RelayFault/1  "RelayFault"

== system APPL_DriverFaultDetection/LogicCtrl/SoftStopPoint ==
  InputSignalBus : Inport
  Bus Creator5 : BusCreator  Inputs=4
  Bus Selector7 : BusSelector  OutputSignals=MotorCmd.MtrCtrlFault_DrHeightMotorCmd,MotorCmd.MtrCtrlFault_DrLengthMotorCmd,MotorCmd.MtrCtrlFault_DrBackMotorCmd,MotorCmd.MtrCtrlFault_DrFrontMotorCmd,SoftStopCnt.MtrCtrlFault_DrMotorSoftStopCntMax,SoftStopCnt.MtrCtrlFault_DrHeightSoftStopCnt,SoftStopCnt.MtrCtrlFault_DrLengthSoftStopCnt,SoftStopCnt.MtrCtrlFault_DrBackSoftStopCnt,SoftStopCnt.MtrCtrlFault_DrFrontSoftStopCnt,StopPosi.MtrCtrlFault_DrHeightStopPosi,StopPosi.MtrCtrlFault_DrLengthStopPosi,StopPosi.MtrCtrlFault_DrBackStopPosi,StopPosi.MtrCtrlFault_DrFrontStopPosi,MotorSize.MtrCtrlFault_DrHeightMotorSize,MotorSize.MtrCtrlFault_DrLengthMotorSize,MotorSize.MtrCtrlFault_DrBackMotorSize,MotorSize.MtrCtrlFault_DrFrontMotorSize,HallCnt.MtrCtrlFault_DrHeightHallCnt,HallCnt.MtrCtrlFault_DrLengthHallCnt,HallCnt.MtrCtrlFault_DrBackHallCnt,HallCnt.MtrCtrlFault_DrFrontHallCnt
  SoftStopPointDetection : Stateflow chart  TreatAsAtomicUnit=on
  SoftStopFault : Outport
  wires:
  Bus Selector7/6 -> SoftStopPointDetection/6(MtrCtrlFault_HeightSoftStopCnt)  "<MtrCtrlFault_DrHeightSoftStopCnt>"
  Bus Selector7/4 -> SoftStopPointDetection/4(MtrCtrlFault_FrontMotorCmd)  "<MtrCtrlFault_DrFrontMotorCmd>"
  Bus Selector7/12 -> SoftStopPointDetection/12(MtrCtrlFault_BackStopPosi)  "<MtrCtrlFault_DrBackStopPosi>"
  Bus Selector7/20 -> SoftStopPointDetection/20(MtrCtrlFault_BackHallCnt)  "<MtrCtrlFault_DrBackHallCnt>"
  SoftStopPointDetection/3(BackSoftStopFault) -> Bus Creator5/3
  InputSignalBus/1 -> Bus Selector7/1
  Bus Selector7/5 -> SoftStopPointDetection/5(MtrCtrlFault_MotorSoftStopCntMax)  "<MtrCtrlFault_DrMotorSoftStopCntMax>"
  Bus Selector7/17 -> SoftStopPointDetection/17(MtrCtrlFault_FrontMotorSize)  "<MtrCtrlFault_DrFrontMotorSize>"
  Bus Selector7/2 -> SoftStopPointDetection/2(MtrCtrlFault_LengthMotorCmd)  "<MtrCtrlFault_DrLengthMotorCmd>"
  Bus Selector7/1 -> SoftStopPointDetection/1(MtrCtrlFault_HeightMotorCmd)  "<MtrCtrlFault_DrHeightMotorCmd>"
  Bus Selector7/10 -> SoftStopPointDetection/10(MtrCtrlFault_HeightStopPosi)  "<MtrCtrlFault_DrHeightStopPosi>"
  Bus Selector7/8 -> SoftStopPointDetection/8(MtrCtrlFault_BackSoftStopCnt)  "<MtrCtrlFault_DrBackSoftStopCnt>"
  Bus Selector7/13 -> SoftStopPointDetection/13(MtrCtrlFault_FrontStopPosi)  "<MtrCtrlFault_DrFrontStopPosi>"
  Bus Selector7/3 -> SoftStopPointDetection/3(MtrCtrlFault_BackMotorCmd)  "<MtrCtrlFault_DrBackMotorCmd>"
  Bus Selector7/9 -> SoftStopPointDetection/9(MtrCtrlFault_FrontSoftStopCnt)  "<MtrCtrlFault_DrFrontSoftStopCnt>"
  SoftStopPointDetection/2(LengthSoftStopFault) -> Bus Creator5/2
  Bus Selector7/14 -> SoftStopPointDetection/14(MtrCtrlFault_HeightMotorSize)  "<MtrCtrlFault_DrHeightMotorSize>"
  SoftStopPointDetection/4(FrontSoftStopFault) -> Bus Creator5/4
  Bus Selector7/15 -> SoftStopPointDetection/15(MtrCtrlFault_LengthMotorSize)  "<MtrCtrlFault_DrLengthMotorSize>"
  Bus Selector7/21 -> SoftStopPointDetection/21(MtrCtrlFault_FrontHallCnt)  "<MtrCtrlFault_DrFrontHallCnt>"
  SoftStopPointDetection/1(HeightSoftStopFault) -> Bus Creator5/1
  Bus Selector7/19 -> SoftStopPointDetection/19(MtrCtrlFault_LengthHallCnt)  "<MtrCtrlFault_DrLengthHallCnt>"
  Bus Selector7/18 -> SoftStopPointDetection/18(MtrCtrlFault_HeightHallCnt)  "<MtrCtrlFault_DrHeightHallCnt>"
  Bus Selector7/7 -> SoftStopPointDetection/7(MtrCtrlFault_LengthSoftStopCnt)  "<MtrCtrlFault_DrLengthSoftStopCnt>"
  Bus Selector7/16 -> SoftStopPointDetection/16(MtrCtrlFault_BackMotorSize)  "<MtrCtrlFault_DrBackMotorSize>"
  Bus Selector7/11 -> SoftStopPointDetection/11(MtrCtrlFault_LengthStopPosi)  "<MtrCtrlFault_DrLengthStopPosi>"
  Bus Creator5/1 -> SoftStopFault/1  "SoftStopFault"

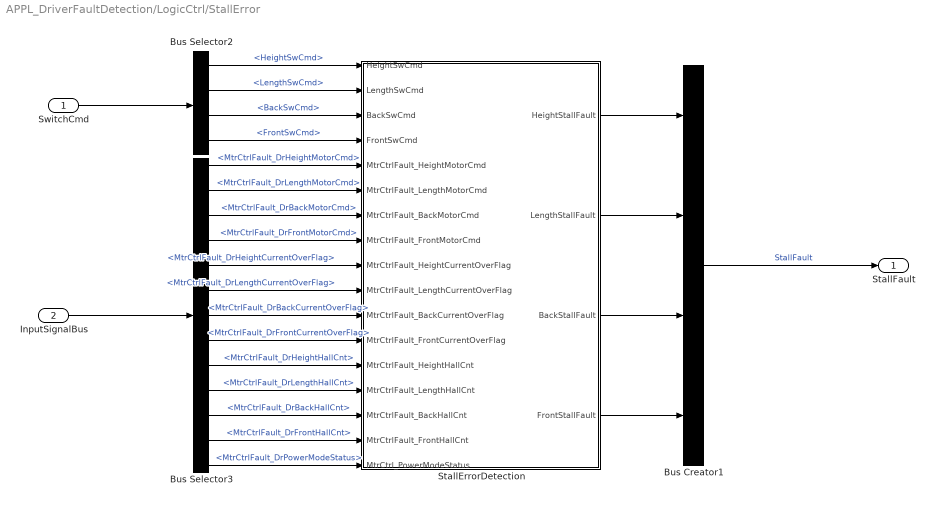
== system APPL_DriverFaultDetection/LogicCtrl/StallError ==
  SwitchCmd : Inport
  InputSignalBus : Inport  Port=2
  Bus Creator1 : BusCreator  Inputs=4
  Bus Selector2 : BusSelector  OutputSignals=HeightSwCmd,LengthSwCmd,BackSwCmd,FrontSwCmd
  Bus Selector3 : BusSelector  OutputSignals=MotorCmd.MtrCtrlFault_DrHeightMotorCmd,MotorCmd.MtrCtrlFault_DrLengthMotorCmd,MotorCmd.MtrCtrlFault_DrBackMotorCmd,MotorCmd.MtrCtrlFault_DrFrontMotorCmd,OverCurrentFlag.MtrCtrlFault_DrHeightCurrentOverFlag,OverCurrentFlag.MtrCtrlFault_DrLengthCurrentOverFlag,OverCurrentFlag.MtrCtrlFault_DrBackCurrentOverFlag,OverCurrentFlag.MtrCtrlFault_DrFrontCurrentOverFlag,HallCnt.MtrCtrlFault_DrHeightHallCnt,HallCnt.MtrCtrlFault_DrLengthHallCnt,HallCnt.MtrCtrlFault_DrBackHallCnt,HallCnt.MtrCtrlFault_DrFrontHallCnt,MtrCtrlFault_DrPowerModeStatus
  StallErrorDetection : Stateflow chart  TreatAsAtomicUnit=on
  StallFault : Outport
  wires:
  Bus Selector3/8 -> StallErrorDetection/12(MtrCtrlFault_FrontCurrentOverFlag)  "<MtrCtrlFault_DrFrontCurrentOverFlag>"
  StallErrorDetection/3(BackStallFault) -> Bus Creator1/3
  Bus Selector3/9 -> StallErrorDetection/13(MtrCtrlFault_HeightHallCnt)  "<MtrCtrlFault_DrHeightHallCnt>"
  Bus Selector2/4 -> StallErrorDetection/4(FrontSwCmd)  "<FrontSwCmd>"
  Bus Selector3/11 -> StallErrorDetection/15(MtrCtrlFault_BackHallCnt)  "<MtrCtrlFault_DrBackHallCnt>"
  Bus Selector3/4 -> StallErrorDetection/8(MtrCtrlFault_FrontMotorCmd)  "<MtrCtrlFault_DrFrontMotorCmd>"
  Bus Selector3/10 -> StallErrorDetection/14(MtrCtrlFault_LengthHallCnt)  "<MtrCtrlFault_DrLengthHallCnt>"
  Bus Selector3/6 -> StallErrorDetection/10(MtrCtrlFault_LengthCurrentOverFlag)  "<MtrCtrlFault_DrLengthCurrentOverFlag>"
  Bus Selector3/3 -> StallErrorDetection/7(MtrCtrlFault_BackMotorCmd)  "<MtrCtrlFault_DrBackMotorCmd>"
  InputSignalBus/1 -> Bus Selector3/1
  Bus Selector3/2 -> StallErrorDetection/6(MtrCtrlFault_LengthMotorCmd)  "<MtrCtrlFault_DrLengthMotorCmd>"
  Bus Selector3/12 -> StallErrorDetection/16(MtrCtrlFault_FrontHallCnt)  "<MtrCtrlFault_DrFrontHallCnt>"
  StallErrorDetection/1(HeightStallFault) -> Bus Creator1/1
  Bus Selector3/1 -> StallErrorDetection/5(MtrCtrlFault_HeightMotorCmd)  "<MtrCtrlFault_DrHeightMotorCmd>"
  Bus Selector2/1 -> StallErrorDetection/1(HeightSwCmd)  "<HeightSwCmd>"
  Bus Selector2/3 -> StallErrorDetection/3(BackSwCmd)  "<BackSwCmd>"
  Bus Selector3/7 -> StallErrorDetection/11(MtrCtrlFault_BackCurrentOverFlag)  "<MtrCtrlFault_DrBackCurrentOverFlag>"
  Bus Selector3/13 -> StallErrorDetection/17(MtrCtrl_PowerModeStatus)  "<MtrCtrlFault_DrPowerModeStatus>"
  StallErrorDetection/2(LengthStallFault) -> Bus Creator1/2
  StallErrorDetection/4(FrontStallFault) -> Bus Creator1/4
  Bus Selector3/5 -> StallErrorDetection/9(MtrCtrlFault_HeightCurrentOverFlag)  "<MtrCtrlFault_DrHeightCurrentOverFlag>"
  Bus Selector2/2 -> StallErrorDetection/2(LengthSwCmd)  "<LengthSwCmd>"
  SwitchCmd/1 -> Bus Selector2/1
  Bus Creator1/1 -> StallFault/1  "StallFault"

== system APPL_DriverFaultDetection/LogicCtrl/SwitchErrDeal ==
  SwitchErrInput : Inport
  " SWProcess " : Stateflow chart  TreatAsAtomicUnit=on
  Bus Creator7 : BusCreator  Inputs=4
  Bus Selector1 : BusSelector  OutputSignals=SwitchCmd.HeightSwCmd,SwitchCmd.LengthSwCmd,SwitchCmd.BackSwCmd,SwitchCmd.FrontSwCmd,RelayFault.HeightMidRelayFault,RelayFault.LengthMidRelayFault,RelayFault.BackMidRelayFault,RelayFault.FrontMidRelayFault,SwAdhesionFault.HeightSwAdhesionFault,SwAdhesionFault.LengthSwAdhesionFault,SwAdhesionFault.BackSwAdhesionFault,SwAdhesionFault.FrontSwAdhesionFault,StallFault.HeightStallFault,StallFault.LengthStallFault,StallFault.BackStallFault,StallFault.FrontStallFault,InputSignalBus.Config.MtrCtrlFault_DrAdjustCfg,InputSignalBus.Config.MtrCtrlFault_DrMemoryCfg,InputSignalBus.MtrCtrlFault_DrPowerModeStatus
  HarSwitchReqOut : Outport
  wires:
  SwitchErrInput/1 -> Bus Selector1/1
  " SWProcess "/2(CurrentLengthSwCmd) -> Bus Creator7/2
  " SWProcess "/3(CurrentBackSwCmd) -> Bus Creator7/3
  " SWProcess "/1(CurrentHeightSwCmd) -> Bus Creator7/1
  " SWProcess "/4(CurrentFrontSwCmd) -> Bus Creator7/4
  Bus Creator7/1 -> HarSwitchReqOut/1  "HarSwitchReq"
  Bus Selector1/1 -> " SWProcess "/1(DrMtr_HeightSwitchCmd)  "<HeightSwCmd>"
  Bus Selector1/2 -> " SWProcess "/2(DrMtr_LengthSwitchCmd)  "<LengthSwCmd>"
  Bus Selector1/3 -> " SWProcess "/3(DrMtr_BackSwitchCmd)  "<BackSwCmd>"
  Bus Selector1/4 -> " SWProcess "/4(DrMtr_FrontSwitchCmd)  "<FrontSwCmd>"
  Bus Selector1/5 -> " SWProcess "/5(DrMtr_HeightRelayAdhesionErr)  "<HeightMidRelayFault>"
  Bus Selector1/6 -> " SWProcess "/6(DrMtr_LengthRelayAdhesionErr)  "<LengthMidRelayFault>"
  Bus Selector1/7 -> " SWProcess "/7(DrMtr_BackRelayAdhesionErr)  "<BackMidRelayFault>"
  Bus Selector1/8 -> " SWProcess "/8(DrMtr_FrontRelayAdhesionErr)  "<FrontMidRelayFault>"
  Bus Selector1/9 -> " SWProcess "/9(DrMtr_HeightSwitchAdheErr)  "<HeightSwAdhesionFault>"
  Bus Selector1/10 -> " SWProcess "/10(DrMtr_LengthSwitchAdheErr)  "<LengthSwAdhesionFault>"
  Bus Selector1/11 -> " SWProcess "/11(DrMtr_BackSwitchAdheErr)  "<BackSwAdhesionFault>"
  Bus Selector1/12 -> " SWProcess "/12(DrMtr_FrontSwitchAdheErr)  "<FrontSwAdhesionFault>"
  Bus Selector1/13 -> " SWProcess "/13(DrMtr_HeightStallErr)  "<HeightStallFault>"
  Bus Selector1/14 -> " SWProcess "/14(DrMtr_LengthStallErr)  "<LengthStallFault>"
  Bus Selector1/15 -> " SWProcess "/15(DrMtr_BackStallErr)  "<BackStallFault>"
  Bus Selector1/16 -> " SWProcess "/16(DrMtr_FrontStallErr)  "<FrontStallFault>"
  Bus Selector1/17 -> " SWProcess "/17(MtrCtrlFault_DrAdjustCfg)  "<MtrCtrlFault_DrAdjustCfg>"
  Bus Selector1/18 -> " SWProcess "/18(MtrCtrlFault_DrMemoryCfg)  "<MtrCtrlFault_DrMemoryCfg>"
  Bus Selector1/19 -> " SWProcess "/19(MtrCtrlFault_PowerModeStatus)  "<MtrCtrlFault_DrPowerModeStatus>"

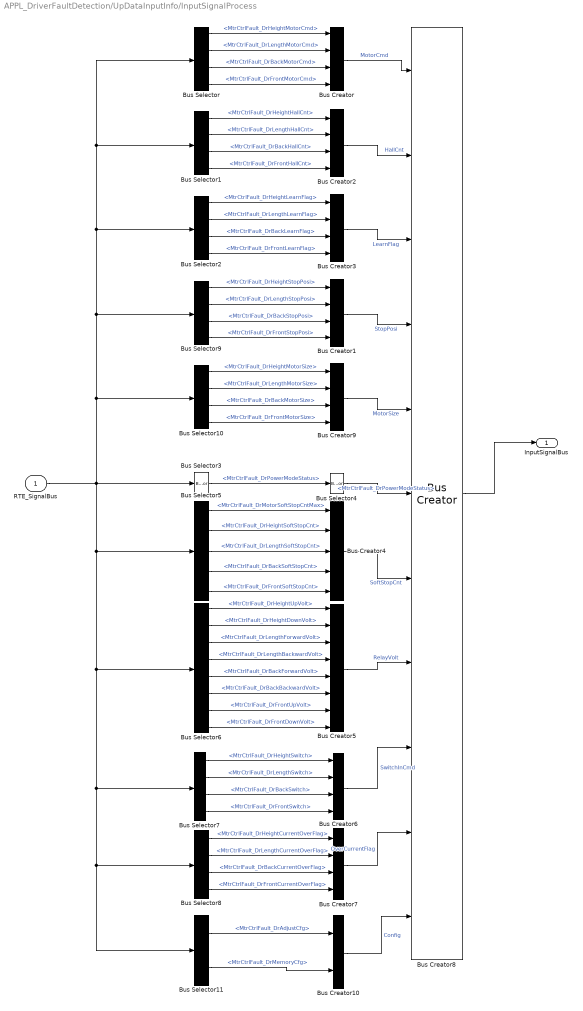
== system APPL_DriverFaultDetection/UpDataInputInfo/InputSignalProcess ==
  RTE_SignalBus : Inport
  Bus Creator{,1..3,6..7,9} (7 alike) : BusCreator  Inputs=4
  Bus Creator10 : BusCreator  Inputs=2
  Bus Creator4 : BusCreator  Inputs=5
  Bus Creator5 : BusCreator  Inputs=8
  Bus Creator8 : BusCreator  Inputs=11
  Bus Selector : BusSelector  OutputSignals=MtrCtrlFault_DrHeightMotorCmd,MtrCtrlFault_DrLengthMotorCmd,MtrCtrlFault_DrBackMotorCmd,MtrCtrlFault_DrFrontMotorCmd
  Bus Selector1 : BusSelector  OutputSignals=MtrCtrlFault_DrHeightHallCnt,MtrCtrlFault_DrLengthHallCnt,MtrCtrlFault_DrBackHallCnt,MtrCtrlFault_DrFrontHallCnt
  Bus Selector10 : BusSelector  OutputSignals=MtrCtrlFault_DrHeightMotorSize,MtrCtrlFault_DrLengthMotorSize,MtrCtrlFault_DrBackMotorSize,MtrCtrlFault_DrFrontMotorSize
  Bus Selector11 : BusSelector  OutputSignals=MtrCtrlFault_DrAdjustCfg,MtrCtrlFault_DrMemoryCfg
  Bus Selector2 : BusSelector  OutputSignals=MtrCtrlFault_DrHeightLearnFlag,MtrCtrlFault_DrLengthLearnFlag,MtrCtrlFault_DrBackLearnFlag,MtrCtrlFault_DrFrontLearnFlag
  Bus Selector3 : BusSelector  OutputSignals=MtrCtrlFault_DrPowerModeStatus
  Bus Selector4 : BusSelector  OutputSignals=MtrCtrlFault_DrPowerModeStatus
  Bus Selector5 : BusSelector  OutputSignals=MtrCtrlFault_DrMotorSoftStopCntMax,MtrCtrlFault_DrHeightSoftStopCnt,MtrCtrlFault_DrLengthSoftStopCnt,MtrCtrlFault_DrBackSoftStopCnt,MtrCtrlFault_DrFrontSoftStopCnt
  Bus Selector6 : BusSelector  OutputSignals=MtrCtrlFault_DrHeightUpVolt,MtrCtrlFault_DrHeightDownVolt,MtrCtrlFault_DrLengthForwardVolt,MtrCtrlFault_DrLengthBackwardVolt,MtrCtrlFault_DrBackForwardVolt,MtrCtrlFault_DrBackBackwardVolt,MtrCtrlFault_DrFrontUpVolt,MtrCtrlFault_DrFrontDownVolt
  Bus Selector7 : BusSelector  OutputSignals=MtrCtrlFault_DrHeightSwitch,MtrCtrlFault_DrLengthSwitch,MtrCtrlFault_DrBackSwitch,MtrCtrlFault_DrFrontSwitch
  Bus Selector8 : BusSelector  OutputSignals=MtrCtrlFault_DrHeightCurrentOverFlag,MtrCtrlFault_DrLengthCurrentOverFlag,MtrCtrlFault_DrBackCurrentOverFlag,MtrCtrlFault_DrFrontCurrentOverFlag
  Bus Selector9 : BusSelector  OutputSignals=MtrCtrlFault_DrHeightStopPosi,MtrCtrlFault_DrLengthStopPosi,MtrCtrlFault_DrBackStopPosi,MtrCtrlFault_DrFrontStopPosi
  InputSignalBus : Outport
  wires:
  Bus Creator8/1 -> InputSignalBus/1
  RTE_SignalBus/1 -> Bus Selector11/1, Bus Selector8/1, Bus Selector7/1, Bus Selector6/1, Bus Selector5/1, Bus Selector3/1, Bus Selector10/1, Bus Selector1/1, Bus Selector/1, Bus Selector2/1, Bus Selector9/1
  Bus Selector/1 -> Bus Creator/1  "<MtrCtrlFault_DrHeightMotorCmd>"
  Bus Selector/2 -> Bus Creator/2  "<MtrCtrlFault_DrLengthMotorCmd>"
  Bus Selector/3 -> Bus Creator/3  "<MtrCtrlFault_DrBackMotorCmd>"
  Bus Selector/4 -> Bus Creator/4  "<MtrCtrlFault_DrFrontMotorCmd>"
  Bus Selector1/2 -> Bus Creator2/2  "<MtrCtrlFault_DrLengthHallCnt>"
  Bus Selector1/1 -> Bus Creator2/1  "<MtrCtrlFault_DrHeightHallCnt>"
  Bus Selector1/3 -> Bus Creator2/3  "<MtrCtrlFault_DrBackHallCnt>"
  Bus Selector1/4 -> Bus Creator2/4  "<MtrCtrlFault_DrFrontHallCnt>"
  Bus Selector2/1 -> Bus Creator3/1  "<MtrCtrlFault_DrHeightLearnFlag>"
  Bus Selector2/2 -> Bus Creator3/2  "<MtrCtrlFault_DrLengthLearnFlag>"
  Bus Selector2/3 -> Bus Creator3/3  "<MtrCtrlFault_DrBackLearnFlag>"
  Bus Selector2/4 -> Bus Creator3/4  "<MtrCtrlFault_DrFrontLearnFlag>"
  Bus Selector3/1 -> Bus Selector4/1  "<MtrCtrlFault_DrPowerModeStatus>"
  Bus Selector5/1 -> Bus Creator4/1  "<MtrCtrlFault_DrMotorSoftStopCntMax>"
  Bus Selector5/2 -> Bus Creator4/2  "<MtrCtrlFault_DrHeightSoftStopCnt>"
  Bus Selector5/3 -> Bus Creator4/3  "<MtrCtrlFault_DrLengthSoftStopCnt>"
  Bus Selector5/4 -> Bus Creator4/4  "<MtrCtrlFault_DrBackSoftStopCnt>"
  Bus Selector5/5 -> Bus Creator4/5  "<MtrCtrlFault_DrFrontSoftStopCnt>"
  Bus Selector6/1 -> Bus Creator5/1  "<MtrCtrlFault_DrHeightUpVolt>"
  Bus Selector6/2 -> Bus Creator5/2  "<MtrCtrlFault_DrHeightDownVolt>"
  Bus Selector6/3 -> Bus Creator5/3  "<MtrCtrlFault_DrLengthForwardVolt>"
  Bus Selector6/4 -> Bus Creator5/4  "<MtrCtrlFault_DrLengthBackwardVolt>"
  Bus Selector6/5 -> Bus Creator5/5  "<MtrCtrlFault_DrBackForwardVolt>"
  Bus Selector6/6 -> Bus Creator5/6  "<MtrCtrlFault_DrBackBackwardVolt>"
  Bus Selector6/7 -> Bus Creator5/7  "<MtrCtrlFault_DrFrontUpVolt>"
  Bus Selector6/8 -> Bus Creator5/8  "<MtrCtrlFault_DrFrontDownVolt>"
  Bus Selector7/1 -> Bus Creator6/1  "<MtrCtrlFault_DrHeightSwitch>"
  Bus Selector7/2 -> Bus Creator6/2  "<MtrCtrlFault_DrLengthSwitch>"
  Bus Selector7/3 -> Bus Creator6/3  "<MtrCtrlFault_DrBackSwitch>"
  Bus Selector7/4 -> Bus Creator6/4  "<MtrCtrlFault_DrFrontSwitch>"
  Bus Selector8/1 -> Bus Creator7/1  "<MtrCtrlFault_DrHeightCurrentOverFlag>"
  Bus Selector8/2 -> Bus Creator7/2  "<MtrCtrlFault_DrLengthCurrentOverFlag>"
  Bus Selector8/3 -> Bus Creator7/3  "<MtrCtrlFault_DrBackCurrentOverFlag>"
  Bus Selector8/4 -> Bus Creator7/4  "<MtrCtrlFault_DrFrontCurrentOverFlag>"
  Bus Creator6/1 -> Bus Creator8/9  "SwitchInCmd"
  Bus Creator7/1 -> Bus Creator8/10  "OverCurrentFlag"
  Bus Creator2/1 -> Bus Creator8/2  "HallCnt"
  Bus Creator5/1 -> Bus Creator8/8  "RelayVolt"
  Bus Creator3/1 -> Bus Creator8/3  "LearnFlag"
  Bus Creator/1 -> Bus Creator8/1  "MotorCmd"
  Bus Creator4/1 -> Bus Creator8/7  "SoftStopCnt"
  Bus Selector4/1 -> Bus Creator8/6  "<MtrCtrlFault_DrPowerModeStatus>"
  Bus Selector9/1 -> Bus Creator1/1  "<MtrCtrlFault_DrHeightStopPosi>"
  Bus Selector9/2 -> Bus Creator1/2  "<MtrCtrlFault_DrLengthStopPosi>"
  Bus Selector9/3 -> Bus Creator1/3  "<MtrCtrlFault_DrBackStopPosi>"
  Bus Selector9/4 -> Bus Creator1/4  "<MtrCtrlFault_DrFrontStopPosi>"
  Bus Creator1/1 -> Bus Creator8/4  "StopPosi"
  Bus Selector10/1 -> Bus Creator9/1  "<MtrCtrlFault_DrHeightMotorSize>"
  Bus Selector10/2 -> Bus Creator9/2  "<MtrCtrlFault_DrLengthMotorSize>"
  Bus Selector10/3 -> Bus Creator9/3  "<MtrCtrlFault_DrBackMotorSize>"
  Bus Selector10/4 -> Bus Creator9/4  "<MtrCtrlFault_DrFrontMotorSize>"
  Bus Creator9/1 -> Bus Creator8/5  "MotorSize"
  Bus Selector11/1 -> Bus Creator10/1  "<MtrCtrlFault_DrAdjustCfg>"
  Bus Selector11/2 -> Bus Creator10/2  "<MtrCtrlFault_DrMemoryCfg>"
  Bus Creator10/1 -> Bus Creator8/11  "Config"
